simulink model "model_vec"  (R2022b)
settings: Solver=ode4  StartTime=0.0  StopTime=1.3  FixedStep=10e-6  RelTol=1e-3
InitFcn:
  | model_
values from neighbouring files (symbols this model uses):
  f = 50    [model_.m]
  i1dn = psi2n/Lm    [model_.m]
  i1qn = sqrt(Inmax^2-i1dn^2)    [model_.m]
  J = 0.4    [model_.m]
  L1 = L1sigma+Lm    (= 0.08477)    [model_.m]
  L1sigma = 2.27e-3    (= 0.00227)    [model_.m]
  L2 = L2sigma+Lm    (= 0.08477)    [model_.m]
  L2sigma = 2.27e-3    (= 0.00227)    [model_.m]
  Lm = 82.5e-3    (= 0.0825)    [model_.m]
  pp = 2    [model_.m]
  psi2n = sqrt(psi2nre^2+psi2nim^2)    [model_.m]
  R1 = 370e-3    (= 0.37)    [model_.m]
  R2 = 225e-3    (= 0.225)    [model_.m]
  R2_vec_model = 225e-3    (= 0.225)    [model_.m]
  sigma = 1-Lm^(2)/(L1*L2)    (= 0.0528396032209)    [model_.m]
  svmFrequency = 10000    [model_.m]
  Us = 400    [model_.m]
libraries: eeTransforms x16, spsMeanLib x7, slpidlib x4, simulink x2, dspsigops x2
(part 2 of 3)

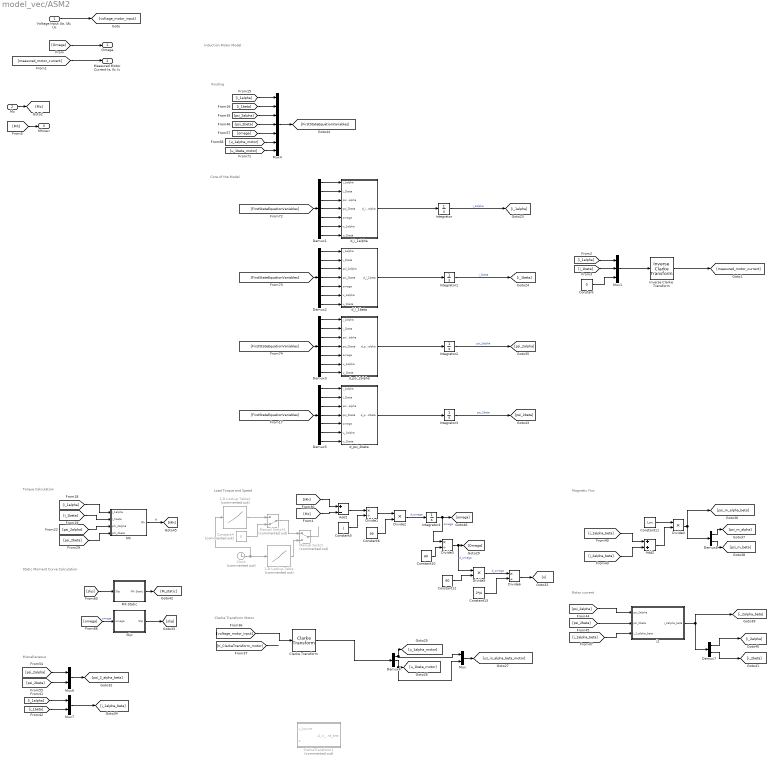
== system model_vec/ASM2 ==
  note: Clarke Transform Motor
  note: Induction Motor Model
  note: Rotor current
  note: Magnetic flux
  note: Static Moment Curve Calculation
  note: Routing
  note: Miscellaneous
  note: Load Torque and Speed
  note: Torque Calculation
  note: Core of the Model
  "Voltage Input Ua, Ub, Uc" : Inport
  Mz : Inport  Port=2
  1-D Lookup Table : Lookup_n-D  Commented=on  NumberOfTableDimensions=1  BreakpointsForDimension1=[0;1.00001;1.001;10]  Table=[0;0;25;25]  InternalRulePriority=Speed  RndMeth=Simplest
  1-D Lookup Table2 : Lookup_n-D  Commented=on  NumberOfTableDimensions=1  BreakpointsForDimension1=[1;2;10]  Table=[0;0;78.48]  InternalRulePriority=Speed  RndMeth=Simplest
  Add1 : Sum  Inputs=+-
  Add2 : Sum
  Clarke Transform : eeTransforms/Clarke Transform  PowerInvariant=off
      settings: LibrarySourceBlock=|
      | ee_sl_lib/Mathematical
      | Transforms/Clarke Transform
  ClarkeTransform1 : Subsystem  Commented=on
  Clock : Clock  Commented=on
  Constant : Constant  Value=0
  Constant10 : Constant  Value=pp
  Constant11 : Constant  Value=Lm
  Constant12 : Constant  Value=60
  Constant13 : Constant  Value=2*pi
  Constant4 : Constant  Commented=on  Value=0
  Constant5 : Constant  Value=J
  Constant6 : Constant  Value=pp
  Demux{1..3,5} (4 alike) : Demux  Outputs=7
  Demux6 : Demux  Outputs=3
  Demux7 : Demux  Outputs=2
  Demux8 : Demux  Outputs=2
  Divide1 : Product  Inputs=*/
  Divide2 : Product  Inputs=**
  Divide3 : Product  Inputs=*/
  Divide4 : Product  Inputs=**
  Divide5 : Product  Inputs=**
  Divide6 : Product  Inputs=*/
  Integrator{,1..4} (5 alike) : Integrator
  Inverse Clarke Transform : eeTransforms/Inverse Clarke Transform  PowerInvariant=off
      settings: LibrarySourceBlock=|
      | ee_sl_lib/Mathematical
      | Transforms/Inverse
      | Clarke Transform
  Manual Switch : ManualSwitch  Commented=on
  Manual Switch1 : ManualSwitch  Commented=on  CurrentSetting=0
  Mh : Subsystem
  Mh Static : Subsystem
  Mux : Mux  Inputs=2
  Mux1 : Mux  Inputs=3
  Mux4 : Mux  Inputs=7
  Mux6 : Mux  Inputs=2
  Mux7 : Mux  Inputs=2
  Slip : Subsystem
  d_i_1alpha : Subsystem
  d_i_1beta : Subsystem
  d_psi_2alpha : Subsystem
  d_psi_2beta : Subsystem
  i2 : Subsystem
  Omega : Outport
  "Measured Motor Current Ia, Ib, Ic" : Outport  Port=2
  Mhnaci : Outport  Port=3
  wires:
  "Voltage Input Ua, Ub, Uc"/1 -> [voltage_motor_input]
  [Omega] -> Omega/1
  [measured_motor_current] -> "Measured Motor Current Ia, Ib, Ic"/1
  Demux1/7 -> d_i_1alpha/7(u_1beta)
  [omega] -> Mux4/5
  Constant6/1 -> Divide2/2
  Demux7/2 -> [i_2beta]
  Constant13/1 -> Divide6/2
  Demux2/3 -> d_i_1beta/3(psi_2alpha)
  [K_ClarkeTransform_motor] -> ?
  1-D Lookup Table2/1 -> Manual Switch1/1
  [i_1alpha_beta] -> i2/3(i_1_alpha_beta)
  d_i_1alpha/1(d_i_1alpha) -> Integrator/1
  Constant4/1 -> Manual Switch1/2
  d_i_1beta/1(d_i_1beta) -> Integrator1/1
  Mh/1(Mh) -> [Mh]  "M"
  Divide6/1 -> [n]
  Demux3/5 -> d_psi_2alpha/5(omega)
  Demux1/2 -> d_i_1alpha/2(i_1beta)
  [i_1alpha] -> Mux7/1
  [psi_2alpha] -> Mh/3(phi_2alpha)
  Demux1/6 -> d_i_1alpha/6(u_1alpha)
  Demux5/7 -> d_psi_2beta/7(u_1beta)
  Demux5/1 -> d_psi_2beta/1(i_1alpha)
  i2/1(i_2alpha_beta) -> Demux7/1, [i_2alpha_beta]
  [i_1beta] -> Mux4/2
  Add2/1 -> Divide4/2
  Slip/1(Slip) -> [slip]
  Demux1/1 -> d_i_1alpha/1(i_1alpha)
  Constant5/1 -> Divide1/2
  Demux3/1 -> d_psi_2alpha/1(i_1alpha)
  Mux4/1 -> [FirstStateEquationVariables]
  [FirstStateEquationVariables] -> Demux5/1
  Integrator4/1 -> Divide3/1, [omega]  "omega"
  Manual Switch1/1 -> Manual Switch/1
  Constant10/1 -> Divide3/2
  Demux3/4 -> d_psi_2alpha/4(psi_2beta)
  Demux7/1 -> [i_2alpha]
  Add1/1 -> Divide1/1
  Demux5/5 -> d_psi_2beta/5(omega)
  [Mh] -> Add1/1
  Demux5/4 -> d_psi_2beta/4(psi_2beta)
  d_psi_2beta/1(d_psi_2beta) -> Integrator3/1
  [u_1beta_motor] -> Mux4/7
  Demux8/1 -> [psi_m_alpha]
  [i_1alpha_beta] -> Add2/1
  [i_1alpha] -> Mh/1(i_1alpha)
  Demux1/5 -> d_i_1alpha/5(omega)
  Demux2/6 -> d_i_1beta/6(u_1alpha)
  Demux2/2 -> d_i_1beta/2(i_1beta)
  Mux7/1 -> [i_1alpha_beta]
  [psi_2beta] -> i2/2(psi_2beta)
  Integrator2/1 -> [psi_2alpha]  "psi_2alpha"
  Demux1/4 -> d_i_1alpha/4(psi_2beta)
  Mux6/1 -> [psi_2_alpha_beta]
  [psi_2beta] -> Mh/4(phi_2beta)
  Constant12/1 -> Divide5/2
  1-D Lookup Table/1 -> Manual Switch/2
  Demux6/2 -> Mux/2, [u_1beta_motor]
  Demux3/3 -> d_psi_2alpha/3(psi_2alpha)
  [psi_2beta] -> Mux4/4
  Demux2/4 -> d_i_1beta/4(psi_2beta)
  [i_1beta] -> Mh/2(i_1beta)
  Divide1/1 -> Divide2/1
  Demux5/6 -> d_psi_2beta/6(u_1alpha)
  Demux2/1 -> d_i_1beta/1(i_1alpha)
  [i_2alpha_beta] -> Add2/2
  d_psi_2alpha/1(d_psi_2alpha) -> Integrator2/1
  Manual Switch/1 -> ?
  Divide2/1 -> Integrator4/1  "d_omega"
  [psi_2beta] -> Mux6/2
  Demux5/2 -> d_psi_2beta/2(i_1beta)
  Demux6/1 -> [u_1alpha_motor], Mux/1
  Divide3/1 -> Divide5/1, [Omega]  "d_omega"
  Integrator1/1 -> [i_1beta]  "i_1beta"
  Integrator3/1 -> [psi_2beta]  "psi_2beta"
  [i_1beta] -> Mux7/2
  Constant11/1 -> Divide4/1
  Demux2/5 -> d_i_1beta/5(omega)
  Demux8/2 -> [psi_m_beta]
  Demux3/6 -> d_psi_2alpha/6(u_1alpha)
  [FirstStateEquationVariables] -> Demux1/1
  Integrator/1 -> [i_1alpha]  "i_1alpha"
  [u_1alpha_motor] -> Mux4/6
  [FirstStateEquationVariables] -> Demux3/1
  [psi_2alpha] -> Mux4/3
  [psi_2alpha] -> i2/1(psi_2alpha)
  Divide5/1 -> Divide6/1  "d_omega"
  Demux2/7 -> d_i_1beta/7(u_1beta)
  Demux3/7 -> d_psi_2alpha/7(u_1beta)
  [slip] -> Mh Static/1(Slip)
  Demux3/2 -> d_psi_2alpha/2(i_1beta)
  Demux1/3 -> d_i_1alpha/3(psi_2alpha)
  [voltage_motor_input] -> Clarke Transform/1
  [FirstStateEquationVariables] -> Demux2/1
  Mh Static/1(Mh Static) -> [M_static]
  [psi_2alpha] -> Mux6/1
  [i_1alpha] -> Mux4/1
  [omega] -> Slip/1(omega)  "omega"
  Clock/1 -> 1-D Lookup Table2/1, 1-D Lookup Table/1
  Demux5/3 -> d_psi_2beta/3(psi_2alpha)
  Divide4/1 -> Demux8/1, [psi_m_alpha_beta]
  Clarke Transform/1 -> Demux6/1
  Mux/1 -> [u1_in_alpha_beta_motor]
  [i_1alpha] -> Mux1/1
  [i_1beta] -> Mux1/2
  Constant/1 -> Mux1/3
  Mux1/1 -> Inverse Clarke Transform/1
  Inverse Clarke Transform/1 -> [measured_motor_current]
  Mz/1 -> [Mz]
  [Mh] -> Mhnaci/1
  [Mz] -> Add1/2

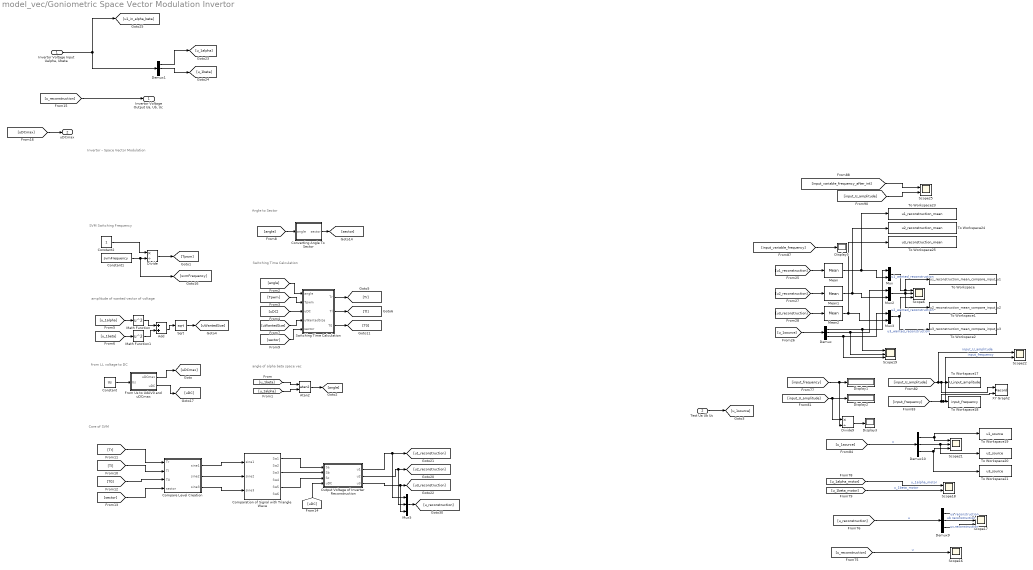
== system model_vec/Goniometric Space Vector Modulation Invertor ==
  note: Invertor – Space Vector Modulation
  note: Core of SVM
  note: Angle to Sector
  note: amplitude of wanted vector of voltage
  note: SVM Switching Frequency
  note: from LL voltage to DC
  note: Switching Time Calculation
  note: angle of alpha beta space vec
  "Invertor Voltage Input Ualpha, Ubeta" : Inport
  Test Ua Ub Uc : Inport  Port=2
  Add : Sum
  Atan2 : Trigonometry  Operator=atan2
  Comparation of Signal with Triangle Wave : Subsystem
  Compare Level Creation : Subsystem
  Constant : Constant  Value=Us
  Constant1 : Constant  Value=svmFrequency
  Constant2 : Constant
  Converting Angle To Sector : MATLAB Function  TreatAsAtomicUnit=on
  Demux{,1,9..10} (4 alike) : Demux  Outputs=3
  Display{1..3,5} (4 alike) : Display
  Divide : Product  Inputs=*/
  Divide9 : Product  Inputs=*/
  From Us to UdAV0 and uDCmax : MATLAB Function  TreatAsAtomicUnit=on
  Math Function : Math  Operator=square
  Math Function1 : Math  Operator=square
  Mean : spsMeanLib/Mean  Freq=svmFrequency  Vinit=0  Ts=0
  Mean1 : spsMeanLib/Mean  Freq=svmFrequency  Vinit=0  Ts=0
  Mean2 : spsMeanLib/Mean  Freq=svmFrequency  Vinit=0  Ts=0
  Mux : Mux  Inputs=2
  Mux2 : Mux  Inputs=2
  Mux3 : Mux  Inputs=2
  Mux5 : Mux  Inputs=3
  Output Voltage of Inverter Reconstruction : Subsystem
  Scope16 : Scope
  Scope{6,17,19,21} (4 alike) : Scope  NumInputPorts=3
  Scope18 : Scope  NumInputPorts=2
  Scope22 : Scope  NumInputPorts=2
  Scope25 : Scope  NumInputPorts=2
  Sqrt : Sqrt
  Switching Time Calculation : MATLAB Function  TreatAsAtomicUnit=on
  To Workspace : ToWorkspace  VariableName=u1_reconstruction_mean_compare_input_u1  SaveFormat=Timeseries  SampleTime=-1
  To Workspace1 : ToWorkspace  VariableName=u2_reconstruction_mean_compare_input_u2  SaveFormat=Timeseries  SampleTime=-1
  To Workspace17 : ToWorkspace  VariableName=U_input_amplitude  SaveFormat=Timeseries  SampleTime=-1
  To Workspace18 : ToWorkspace  VariableName=input_frequency  SaveFormat=Timeseries  SampleTime=-1
  To Workspace19 : ToWorkspace  VariableName=u1_source  SaveFormat=Timeseries  SampleTime=-1
  To Workspace2 : ToWorkspace  VariableName=u3_reconstruction_mean_compare_input_u3  SaveFormat=Timeseries  SampleTime=-1
  To Workspace20 : ToWorkspace  VariableName=u2_source  SaveFormat=Timeseries  SampleTime=-1
  To Workspace21 : ToWorkspace  VariableName=u3_source  SaveFormat=Timeseries  SampleTime=-1
  To Workspace23 : ToWorkspace  VariableName=u1_reconstruction_mean  SaveFormat=Timeseries  SampleTime=-1
  To Workspace24 : ToWorkspace  VariableName=u2_reconstruction_mean  SaveFormat=Timeseries  SampleTime=-1
  To Workspace25 : ToWorkspace  VariableName=u3_reconstruction_mean  SaveFormat=Timeseries  SampleTime=-1
  XY Graph2 : Record  FileSettingsInternal="{\"entries\":[{\"content\":{\"excelSettings\":{\"content\":{},\"type\":\"Streamout.ExcelSettings\"}},\"type\":\"Streamout.FileSettingStorage\",\"uuid\":\"02ea5c6f-de8f-4b43-b0a6-6bc7c7bf4af1\"}],\"packageUris\":[\"http://schema.mathworks.com/mf0/streamout_blocks/R2020a\"],\"version\":\"1.0\"}"  Layout=[1 1]  SignalsInternal="{\"entries\":[{\"content\":{\"signals\":[{\"content\":{\"blockPath\":[\"model_vec/Goniometric Space Vector Modulation Invertor/XY Graph2\"],\"channel\":[],\"dimensions\":[1],\"domain\":\"model_vec/Goniometric Space Vector Modulation Invertor/XY Graph2\",\"lineColor\":\"#0072bd\",\"plots\":[],\"port\":1,\"sid\":[\"\"],\"signalID\":2164,\"signalName\":\"input_U_amplitude\"},\"type\":\"RecordBlkView.Signal\",\"uuid\":\"30d02a87-ee14-4616-b6b9-5fcb510cce3f\"},{\"content\":{\"blockPath\":[\"model_vec/Goniometric Space Vector Modulation Invertor/XY Graph2\"],\"channel\":[],\"dimensions\":[1],\"domain\":\"model_vec/Goniometric Space Vector Modulation Invertor/XY Graph2\",\"lineColor\":\"#d95319\",\"plots\":[],\"port\":2,\"sid\":[\"\"],\"signalID\":2168,\"signalName\":\"input_frequency\"},\"type\":\"RecordBlkView.Signal\",\"uuid\":\"35793a4a-81a6-485c-847a-b82e39ee9c73\"}]},\"type\":\"RecordBlkView.InputSignals\",\"uuid\":\"5b8892b0-9142-4253-8381-be57873c5d0a\"}],\"packageUris\":[\"http://schema.mathworks.com/mf0/streamout_blocks/R2020a\"],\"version\":\"1.0\"}"  VisualizationBindings="{\"xyplotplugin\":{\"info\":[{\"series\":[],\"subplotID\":1}]}}"  CompatibilityTag=XY
  "Invertor Voltage Output Ua, Ub, Uc" : Outport
  uDCmax : Outport  Port=2
  wires:
  "Invertor Voltage Input Ualpha, Ubeta"/1 -> Demux1/1, [u1_in_alpha_beta]
  [u_reconstruction] -> "Invertor Voltage Output Ua, Ub, Uc"/1
  Demux1/1 -> [u_1alpha]
  Demux1/2 -> [u_1beta]
  [uDCmax] -> uDCmax/1
  Output Voltage of Inverter Reconstruction/3(u3) -> Mux5/3, [u3_reconstruction]
  [u_1beta] -> Atan2/1
  From Us to UdAV0 and uDCmax/1(uDCmax) -> [uDCmax]
  Divide/1 -> [Tpwm]
  [angle] -> Switching Time Calculation/1(angle)
  Converting Angle To Sector/1(sector) -> [sector]
  Atan2/1 -> [angle]
  [angle] -> Converting Angle To Sector/1(angle)
  Constant1/1 -> [svmFrequency], Divide/2
  [sector] -> Compare Level Creation/4(sector)
  Math Function/1 -> Add/1
  [Tr] -> Compare Level Creation/1(Tr)
  [uDC] -> Output Voltage of Inverter Reconstruction/4(uDC)
  [u_1alpha] -> Math Function/1
  [u_1alpha] -> Atan2/2
  [Tl] -> Compare Level Creation/2(Tl)
  Add/1 -> Sqrt/1
  [sector] -> Switching Time Calculation/5(sector)
  Constant/1 -> From Us to UdAV0 and uDCmax/1(Us)
  Output Voltage of Inverter Reconstruction/2(u2) -> Mux5/2, [u2_reconstruction]
  [Tpwm] -> Switching Time Calculation/2(Tpwm)
  Compare Level Creation/3(sine3) -> Comparation of Signal with Triangle Wave/3(sine3)
  Switching Time Calculation/3(T0) -> [T0]
  Comparation of Signal with Triangle Wave/3(Sw3) -> Output Voltage of Inverter Reconstruction/2(Sb)
  Comparation of Signal with Triangle Wave/5(Sw5) -> Output Voltage of Inverter Reconstruction/3(Sc)
  Output Voltage of Inverter Reconstruction/1(u1) -> Mux5/1, [u1_reconstruction]
  Compare Level Creation/1(sine1) -> Comparation of Signal with Triangle Wave/1(sine1)
  [uDC] -> Switching Time Calculation/3(uDC)
  Mux5/1 -> [u_reconstruction]
  From Us to UdAV0 and uDCmax/2(uDC) -> [uDC]
  [u_1beta] -> Math Function1/1
  Comparation of Signal with Triangle Wave/1(Sw1) -> Output Voltage of Inverter Reconstruction/1(Sa)
  Compare Level Creation/2(sine2) -> Comparation of Signal with Triangle Wave/2(sine2)
  Constant2/1 -> Divide/1
  Math Function1/1 -> Add/2
  [uWantedSize] -> Switching Time Calculation/4(uWantedSize)
  Switching Time Calculation/1(Tr) -> [Tr]
  Sqrt/1 -> [uWantedSize]
  [T0] -> Compare Level Creation/3(T0)
  Switching Time Calculation/2(Tl) -> [Tl]
  Divide9/1 -> Display3/1
  Mux3/1 -> Scope6/3, To Workspace2/1  "u3_wanted_reconstruction"
  [input_variable_frequency_after_int] -> Scope25/1
  [input_U_amplitude] -> Scope25/2
  Demux10/2 -> To Workspace20/1, Scope21/2
  Demux/1 -> Scope19/1, Mux/1
  [u_reconstruction] -> Demux9/1  "u"
  Mean2/1 -> To Workspace25/1, Mux3/2
  Demux10/3 -> To Workspace21/1, Scope21/3
  Demux/3 -> Scope19/3, Mux3/1
  Demux10/1 -> Scope21/1, To Workspace19/1
  [input_frequency] -> Scope22/2, To Workspace18/1, XY Graph2/2  "input_frequency"
  Demux/2 -> Scope19/2, Mux2/1
  [input_U_amplitude] -> Divide9/1, Display2/1
  [input_U_amplitude] -> Scope22/1, XY Graph2/1, To Workspace17/1  "input_U_amplitude"
  [u_1source] -> Demux10/1  "u"
  Mux/1 -> Scope6/1, To Workspace/1  "u1_wanted_reconstruction"
  Mean/1 -> To Workspace23/1, Mux/2
  [input_variable_frequency] -> Display5/1
  [u1_reconstruction] -> Mean/1
  [u3_reconstruction] -> Mean2/1
  Mux2/1 -> Scope6/2, To Workspace1/1  "u2_wanted_reconstruction"
  Mean1/1 -> To Workspace24/1, Mux2/2
  [input_frequency] -> Divide9/2, Display1/1
  [u2_reconstruction] -> Mean1/1
  Demux9/2 -> Scope17/2  "ub reconstruction"
  [u_reconstruction] -> Scope16/1  "u"
  [u_1alpha_motor] -> Scope18/1  "u_1alpha_motor"
  [u_1beta_motor] -> Scope18/2  "u_1beta_motor"
  [u_1source] -> Demux/1
  Demux9/1 -> Scope17/1  "ua reconstruction"
  Demux9/3 -> Scope17/3  "uc reconstruction"
  Test Ua Ub Uc/1 -> [u_1source]

== system model_vec/I-n model ==
  "Measured Motor Current Ia, Ib, Ic" : Inport
  Omega : Inport  Port=2
  Add : Sum  Inputs=+--
  Add1 : Sum  Inputs=+-+
  Atan2 : Trigonometry  Operator=atan2
  Clarke Transform : eeTransforms/Clarke Transform  PowerInvariant=off
      settings: LibrarySourceBlock=|
      | ee_sl_lib/Mathematical
      | Transforms/Clarke Transform
  Constant10 : Constant  Value=Lm
  Constant{7,9,11..12} (4 alike) : Constant  Value=L2
  Constant{2,5,13..14} (4 alike) : Constant  Value=R2_vec_model
  Constant4 : Constant  Value=pp
  Constant8 : Constant  Value=Lm
  Demux : Demux  Outputs=3
  Divide{,1..6} (7 alike) : Product  Inputs=**
  Divide10 : Product  Inputs=*/
  Divide7 : Product  Inputs=*/
  Divide8 : Product  Inputs=**/
  Divide9 : Product  Inputs=**/
  Integrator : Integrator
  Integrator1 : Integrator
  Module of Vector1 : Subsystem
  Mux : Mux  Inputs=2
  Theta : Outport
  Psi_2_module : Outport  Port=2
  Psi_2_alpha_beta : Outport  Port=3
  wires:
  "Measured Motor Current Ia, Ib, Ic"/1 -> Clarke Transform/1
  Clarke Transform/1 -> Demux/1
  Integrator1/1 -> [Psi_2_beta]  "Psi2beta"
  Demux/1 -> Divide/1  "i_1_alpha"
  Demux/2 -> Divide3/1  "i_1_beta"
  [omega] -> Divide2/1
  Integrator/1 -> [Psi_2_alpha]  "Psi2alpha"
  [Psi_2_beta] -> Divide2/2
  [Psi_2_alpha] -> Divide1/1
  Divide/1 -> Add/1
  Divide1/1 -> Add/2
  Divide2/1 -> Add/3
  Add/1 -> Integrator/1
  [Psi_2_beta] -> Divide4/1
  [Psi_2_alpha] -> Divide5/2
  [omega] -> Divide5/1
  Divide3/1 -> Add1/1
  Divide4/1 -> Add1/2
  Divide5/1 -> Add1/3
  Add1/1 -> Integrator1/1
  [Psi_2_beta] -> Atan2/1
  [Psi_2_alpha] -> Atan2/2
  Atan2/1 -> Theta/1
  [Psi_2_alpha] -> Mux/1, Module of Vector1/1(In1)
  [Psi_2_beta] -> Mux/2, Module of Vector1/2(In2)
  Module of Vector1/1(Psi) -> Psi_2_module/1  "psi_2_module"
  Omega/1 -> Divide6/1
  Constant4/1 -> Divide6/2
  Divide6/1 -> [omega]
  Mux/1 -> Psi_2_alpha_beta/1
  Divide7/1 -> Divide1/2
  Constant13/1 -> Divide7/1
  Constant7/1 -> Divide7/2
  Constant8/1 -> Divide8/1
  Constant5/1 -> Divide8/2
  Constant9/1 -> Divide8/3
  Divide8/1 -> Divide/2
  Constant11/1 -> Divide9/3
  Constant14/1 -> Divide9/2
  Constant10/1 -> Divide9/1
  Divide9/1 -> Divide3/2
  Constant12/1 -> Divide10/2
  Constant2/1 -> Divide10/1
  Divide10/1 -> Divide4/2

== system model_vec/Inverse Park1 ==
  dq0 : Inport
  Theta : Inport  Port=2
  Add : Sum  Inputs=+-
  Add1 : Sum
  Constant : Constant  Value=0
  Cos : Trigonometry  Operator=cos
  Cos1 : Trigonometry  Operator=cos
  Demux : Demux  Outputs=3
  Divide{,1..3} (4 alike) : Product  Inputs=**
  Mux : Mux  Inputs=3
  Sin : Trigonometry
  Sin1 : Trigonometry
  alpha_beta_0 : Outport
  wires:
  Constant/1 -> Mux/3
  Mux/1 -> alpha_beta_0/1
  Add1/1 -> Mux/2
  Add/1 -> Mux/1
  Divide2/1 -> Add1/2
  Divide3/1 -> Add1/1
  Divide/1 -> Add/2
  Divide1/1 -> Add/1
  [Theta] -> Cos1/1
  [Theta] -> Sin1/1
  Sin1/1 -> Divide2/1
  Cos1/1 -> Divide3/1
  [q] -> Divide3/2
  [d] -> Divide2/2
  [q] -> Divide/2
  [d] -> Divide1/2
  Demux/2 -> [q]
  Demux/1 -> [d]
  Cos/1 -> Divide1/1
  Sin/1 -> Divide/1
  [Theta] -> Sin/1
  [Theta] -> Cos/1
  Theta/1 -> [Theta]
  dq0/1 -> Demux/1

== system model_vec/Min-Max Method Space Vector Modulation Invertor ==
  note: from LL voltage to DC
  Ua Ub Uc : Inport
  Add12 : Sum
  Add13 : Sum  Inputs=+-
  Add14 : Sum  Inputs=+-
  Add15 : Sum  Inputs=+-
  Comparation of Signal with Triangle Wave : Subsystem
  Constant : Constant  Value=Us
  Constant13 : Constant  Value=270
  Constant14 : Constant  Value=2
  Demux : Demux  Outputs=3
  Demux1 : Demux  Outputs=3
  Divide{1..2,10..11} (4 alike) : Product  Inputs=*/
  From Us to UdAV0 and uDCmax : MATLAB Function  TreatAsAtomicUnit=on
  Max2 : MinMax  Function=max
  Max3 : MinMax
  Mean : spsMeanLib/Mean  Freq=svmFrequency  Vinit=0  Ts=0
  Mean1 : spsMeanLib/Mean  Freq=svmFrequency  Vinit=0  Ts=0
  Mean2 : spsMeanLib/Mean  Freq=svmFrequency  Vinit=0  Ts=0
  Mux : Mux  Inputs=2
  Mux2 : Mux  Inputs=2
  Mux3 : Mux  Inputs=2
  Mux5 : Mux  Inputs=3
  Output Voltage of Inverter Reconstruction : Subsystem
  Scope1 : Scope  NumInputPorts=3
  Scope6 : Scope  NumInputPorts=3
  u_reconstruction : Outport
  wires:
  Max2/1 -> Add12/1
  Ua Ub Uc/1 -> Demux1/1, Demux/1, Max3/1, Max2/1
  Constant13/1 -> Divide2/2, Divide1/2, Divide11/2
  Add13/1 -> Divide11/1
  Max3/1 -> Add12/2
  Add12/1 -> Divide10/1
  Constant14/1 -> Divide10/2
  Divide10/1 -> Add15/2, Add13/2, Add14/2
  Demux/1 -> Add13/1
  Comparation of Signal with Triangle Wave/5(Sw5) -> Output Voltage of Inverter Reconstruction/3(Sc)
  From Us to UdAV0 and uDCmax/2(uDC) -> [uDC]
  Output Voltage of Inverter Reconstruction/1(u1) -> Mean/1, Mux5/1, [u1_reconstruction]
  Output Voltage of Inverter Reconstruction/2(u2) -> Mean1/1, Mux5/2, [u2_reconstruction]
  [uDC] -> Output Voltage of Inverter Reconstruction/4(uDC)
  Mux5/1 -> u_reconstruction/1
  From Us to UdAV0 and uDCmax/1(uDCmax) -> [uDCmax]
  Comparation of Signal with Triangle Wave/1(Sw1) -> Output Voltage of Inverter Reconstruction/1(Sa)
  Output Voltage of Inverter Reconstruction/3(u3) -> Mean2/1, Mux5/3, [u3_reconstruction]
  Constant/1 -> From Us to UdAV0 and uDCmax/1(Us)
  Comparation of Signal with Triangle Wave/3(Sw3) -> Output Voltage of Inverter Reconstruction/2(Sb)
  Demux/2 -> Add14/1
  Demux/3 -> Add15/1
  Divide11/1 -> Comparation of Signal with Triangle Wave/1(sine1), Scope6/1
  Add14/1 -> Divide1/1
  Add15/1 -> Divide2/1
  Divide1/1 -> Comparation of Signal with Triangle Wave/2(sine2), Scope6/2
  Divide2/1 -> Scope6/3, Comparation of Signal with Triangle Wave/3(sine3)
  Mean/1 -> Mux/1
  Mean1/1 -> Mux2/1
  Mean2/1 -> Mux3/1
  Mux/1 -> Scope1/1  "u1_wanted_reconstruction"
  Mux2/1 -> Scope1/2  "u2_wanted_reconstruction"
  Mux3/1 -> Scope1/3  "u3_wanted_reconstruction"
  Demux1/3 -> Mux3/2
  Demux1/2 -> Mux2/2
  Demux1/1 -> Mux/2

== system model_vec/Odvazbeni u1d (pricist k u1d) (minusy jsou uvnitr) ==
  i1q : Inport
  psi2d : Inport  Port=2
  omega_s : Inport  Port=3
  Add11 : Sum  Inputs=+-
  Add14 : Sum  Inputs=--
  Constant3 : Constant  Value=L1
  Constant5 : Constant  Value=Lm^2/L2
  Constant6 : Constant  Value=Lm*R2_vec_model/L2^2
  Divide : Product  Inputs=***
  Divide1 : Product  Inputs=**
  odvazbeni : Outport
  wires:
  Constant6/1 -> Divide1/1
  i1q/1 -> Divide/3
  Divide/1 -> Add14/1
  Add11/1 -> Divide/1
  psi2d/1 -> Divide1/2
  Constant5/1 -> Add11/2
  Add14/1 -> odvazbeni/1
  Constant3/1 -> Add11/1
  Divide1/1 -> Add14/2
  omega_s/1 -> Divide/2

== system model_vec/Odvazbeni u1q (pricist k u1q) (minusy jsou uvnitr) ==
  i1d : Inport
  psi2d : Inport  Port=2
  omega_s : Inport  Port=3
  Add11 : Sum  Inputs=+-
  Add14 : Sum
  Constant1 : Constant  Value=2*pi*f
  Constant2 : Constant  Value=Lm/L2
  Constant3 : Constant  Value=L1
  Constant5 : Constant  Value=Lm^2/L2
  Divide : Product  Inputs=***
  Divide1 : Product  Inputs=***
  odvazbeni : Outport
  wires:
  Divide1/1 -> Add14/2
  Constant3/1 -> Add11/1
  Add14/1 -> odvazbeni/1
  Constant5/1 -> Add11/2
  psi2d/1 -> Divide1/2
  Add11/1 -> Divide/1
  Divide/1 -> Add14/1
  i1d/1 -> Divide/3
  Constant1/1 -> Divide1/1
  Constant2/1 -> Divide1/3
  omega_s/1 -> Divide/2

== system model_vec/Omega*Time Calculation1 ==
  frequency : Inport
  Clock : Clock  Commented=on
  Constant1 : Constant  Commented=on  Value=50
  Constant2 : Constant  Commented=on
  Constant4 : Constant  Value=2
  Constant5 : Constant  Value=pi
  Divide1 : Product  Inputs=***
  Equal : RelationalOperator  Commented=on  OutDataTypeStr=boolean  RndMeth=Simplest  InputSameDT=off
  Switch : Switch  Commented=on  Criteria=u2 > Threshold  SaturateOnIntegerOverflow=off  InputSameDT=off
  omega_t : Outport
  wires:
  Divide1/1 -> omega_t/1
  frequency/1 -> Divide1/3
  Constant5/1 -> Divide1/2
  Clock/1 -> Switch/1
  Constant4/1 -> Divide1/1
  Constant1/1 -> Equal/2
  Equal/1 -> Switch/2
  Constant2/1 -> Switch/3

== system model_vec/Triggered Subsystem ==
  In1 : Inport
  Trigger : TriggerPort  VariantControl=(inherit)
  Out1 : Outport
  wires:
  In1/1 -> Out1/1

== system model_vec/u4 ==
  amplitude : Inport
  omega_t : Inport  Port=2
  Add4 : Sum
  Constant6 : Constant  Value=0
  Divide3 : Product  Inputs=**
  Sin : Trigonometry
  u1 : Outport
  wires:
  Divide3/1 -> u1/1
  Sin/1 -> Divide3/1
  Add4/1 -> Sin/1
  Constant6/1 -> Add4/2
  omega_t/1 -> Add4/1
  amplitude/1 -> Divide3/2

== system model_vec/u5 ==
  amplitude : Inport
  omega_t : Inport  Port=2
  Add4 : Sum
  Constant6 : Constant  Value=(2*pi/3)
  Divide3 : Product  Inputs=**
  Sin : Trigonometry
  u2 : Outport
  wires:
  omega_t/1 -> Add4/1
  Constant6/1 -> Add4/2
  Add4/1 -> Sin/1
  Sin/1 -> Divide3/1
  Divide3/1 -> u2/1
  amplitude/1 -> Divide3/2

== system model_vec/u6 ==
  amplitude : Inport
  omega_t : Inport  Port=2
  Add4 : Sum
  Constant6 : Constant  Value=(-2*pi/3)
  Divide3 : Product  Inputs=**
  Sin : Trigonometry
  u3 : Outport
  wires:
  Divide3/1 -> u3/1
  amplitude/1 -> Divide3/2
  Sin/1 -> Divide3/1
  Add4/1 -> Sin/1
  Constant6/1 -> Add4/2
  omega_t/1 -> Add4/1

== system model_vec/ASM/ClarkeTransform1 ==
  u_1source : Inport
  K : Inport  Port=2
  Add1 : Sum  Inputs=+++
  Add2 : Sum  Inputs=+++
  Demux4 : Demux  Outputs=3
  Demux5 : Demux  Outputs=3
  Divide2 : Product  Inputs=**
  Divide3 : Product  Inputs=**
  Gain : Gain  Gain=-1/2
  Gain1 : Gain  Gain=-1/2
  Gain2 : Gain  Gain=-sqrt(3)/2
  Gain3 : Gain  Gain=sqrt(3)/2
  Gain4 : Gain
  Gain5 : Gain  Gain=0
  Mux2 : Mux  Inputs=2
  u1_in_alpha_beta : Outport
  wires:
  Demux4/1 -> Gain4/1  "ua"
  Divide2/1 -> Mux2/1  "u_1alpha"
  [K_ClarkeTransform] -> Divide2/2
  Add1/1 -> Divide2/1
  Demux4/2 -> Gain/1  "ub"
  Divide3/1 -> Mux2/2  "u_1beta"
  Gain5/1 -> Add2/1
  Gain/1 -> Add1/2
  Demux5/1 -> Gain5/1  "ua"
  Gain3/1 -> Add2/3
  [K_ClarkeTransform] -> Divide3/2
  Gain2/1 -> Add2/2
  Gain1/1 -> Add1/3
  Demux5/2 -> Gain2/1  "ub"
  Demux5/3 -> Gain3/1  "uc"
  Add2/1 -> Divide3/1
  Gain4/1 -> Add1/1
  u_1source/1 -> Demux5/1, Demux4/1
  K/1 -> [K_ClarkeTransform]
  Mux2/1 -> u1_in_alpha_beta/1
  Demux4/3 -> Gain1/1  "uc"

== system model_vec/ASM/Mh ==
  i_1alpha : Inport
  i_1beta : Inport  Port=2
  phi_2alpha : Inport  Port=3
  phi_2beta : Inport  Port=4
  Add : Sum  Inputs=+-
  Constant : Constant  Value=3/2
  Constant1 : Constant  Value=pp
  Constant2 : Constant  Value=Lm
  Constant3 : Constant  Value=L2
  Divide{,1,3..5} (5 alike) : Product  Inputs=**
  Divide2 : Product  Inputs=*/
  Mh : Outport
  wires:
  Constant/1 -> Divide/1
  Constant1/1 -> Divide/2
  Divide/1 -> Divide1/1
  Constant2/1 -> Divide2/1
  Constant3/1 -> Divide2/2
  Divide2/1 -> Divide1/2
  Divide1/1 -> Divide3/2
  phi_2alpha/1 -> Divide4/2
  i_1beta/1 -> Divide4/1
  Divide4/1 -> Add/1
  phi_2beta/1 -> Divide5/1
  i_1alpha/1 -> Divide5/2
  Divide5/1 -> Add/2
  Add/1 -> Divide3/1
  Divide3/1 -> Mh/1

== system model_vec/ASM/Mh Static ==
  Slip : Inport
  Add3 : Sum
  Add4 : Sum
  Add6 : Sum
  Constant10 : Constant  Value=230^(2)
  Constant11 : Constant  Value=pp
  Constant14 : Constant  Value=2*pi*f
  Constant15 : Constant  Value=R1
  Constant16 : Constant  Value=R2
  Constant21 : Constant  Value=2*pi*f
  Constant22 : Constant  Value=L1sigma
  Constant23 : Constant  Value=L2sigma
  Constant8 : Constant  Value=3
  Constant9 : Constant  Value=R2
  Divide10 : Product  Inputs=/*
  Divide11 : Product  Inputs=*/
  Divide15 : Product  Inputs=**
  Divide6 : Product  Inputs=****
  Divide7 : Product  Inputs=*/
  Divide8 : Product  Inputs=**
  Math Function : Math  Operator=square
  Math Function2 : Math  Operator=square
  Reprezentace s s*omega1*L2sigma : Subsystem
  Mh Static : Outport
  wires:
  Slip/1 -> Divide8/2, Divide11/2
  Constant11/1 -> Divide6/4
  Constant10/1 -> Divide6/3
  Add4/1 -> Math Function/1
  Constant16/1 -> Divide11/1
  Constant9/1 -> Divide6/2
  Constant23/1 -> Add6/2
  Constant15/1 -> Add4/1
  Divide15/1 -> Math Function2/1
  Divide8/1 -> Divide7/2
  Constant14/1 -> Divide8/1
  Math Function/1 -> Add3/1
  Divide7/1 -> Divide10/2
  Divide10/1 -> Mh Static/1
  Divide11/1 -> Add4/2
  Constant22/1 -> Add6/1
  Add6/1 -> Divide15/1
  Constant8/1 -> Divide6/1
  Constant21/1 -> Divide15/2
  Add3/1 -> Divide10/1
  Divide6/1 -> Divide7/1
  Math Function2/1 -> Add3/2

== system model_vec/ASM/Module of Vector ==
  In1 : Inport
  In2 : Inport  Port=2
  Add2 : Sum
  Math Function : Math  Operator=square
  Math Function1 : Math  Operator=square
  Sqrt : Sqrt
  Out1 : Outport
  wires:
  In1/1 -> Math Function/1
  Sqrt/1 -> Out1/1
  Math Function/1 -> Add2/1
  Math Function1/1 -> Add2/2
  In2/1 -> Math Function1/1
  Add2/1 -> Sqrt/1

== system model_vec/ASM/Module of Vector1 ==
  In1 : Inport
  In2 : Inport  Port=2
  Add2 : Sum
  Math Function : Math  Operator=square
  Math Function1 : Math  Operator=square
  Sqrt : Sqrt
  Out1 : Outport
  wires:
  Add2/1 -> Sqrt/1
  In2/1 -> Math Function1/1
  Math Function1/1 -> Add2/2
  Math Function/1 -> Add2/1
  Sqrt/1 -> Out1/1
  In1/1 -> Math Function/1

== system model_vec/ASM/Module of Vector2 ==
  In1 : Inport
  In2 : Inport  Port=2
  Add2 : Sum
  Math Function : Math  Operator=square
  Math Function1 : Math  Operator=square
  Sqrt : Sqrt
  Out1 : Outport
  wires:
  Add2/1 -> Sqrt/1
  In2/1 -> Math Function1/1
  Math Function1/1 -> Add2/2
  Math Function/1 -> Add2/1
  Sqrt/1 -> Out1/1
  In1/1 -> Math Function/1

== system model_vec/ASM/Slip ==
  omega : Inport
  Add2 : Sum  Inputs=+-
  Constant12 : Constant  Value=2*pi*f
  Constant13 : Constant  Value=2*pi*f
  Divide9 : Product  Inputs=*/
  Slip : Outport
  wires:
  omega/1 -> Add2/2  "Omega"
  Divide9/1 -> Slip/1
  Constant12/1 -> Add2/1
  Add2/1 -> Divide9/1
  Constant13/1 -> Divide9/2

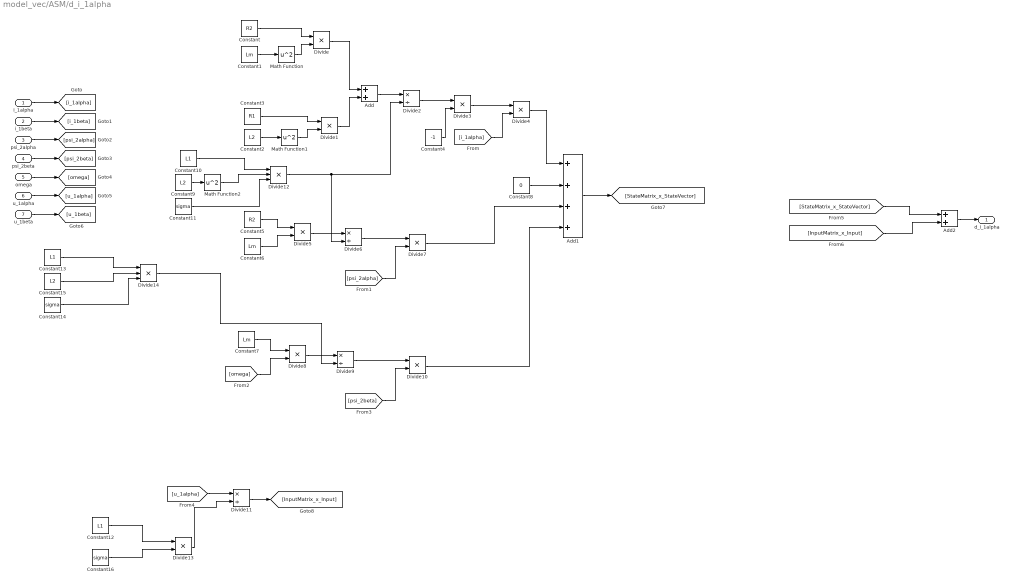
== system model_vec/ASM/d_i_1alpha ==
  i_1alpha : Inport
  i_1beta : Inport  Port=2
  psi_2alpha : Inport  Port=3
  psi_2beta : Inport  Port=4
  omega : Inport  Port=5
  u_1alpha : Inport  Port=6
  u_1beta : Inport  Port=7
  Add : Sum
  Add1 : Sum  Inputs=++++
  Add2 : Sum
  Constant : Constant  Value=R2
  Constant1 : Constant  Value=Lm
  Constant10 : Constant  Value=L1
  Constant11 : Constant  Value=sigma
  Constant12 : Constant  Value=L1
  Constant13 : Constant  Value=L1
  Constant14 : Constant  Value=sigma
  Constant15 : Constant  Value=L2
  Constant16 : Constant  Value=sigma
  Constant2 : Constant  Value=L2
  Constant3 : Constant  Value=R1
  Constant4 : Constant  Value=-1
  Constant5 : Constant  Value=R2
  Constant6 : Constant  Value=Lm
  Constant7 : Constant  Value=Lm
  Constant8 : Constant  Value=0
  Constant9 : Constant  Value=L2
  Divide{,1,3..5,7..8,10,13} (9 alike) : Product  Inputs=**
  Divide{2,6,9,11} (4 alike) : Product  Inputs=*/
  Divide12 : Product  Inputs=***
  Divide14 : Product  Inputs=***
  Math Function : Math  Operator=square
  Math Function1 : Math  Operator=square
  Math Function2 : Math  Operator=square
  d_i_1alpha : Outport
  wires:
  Constant1/1 -> Math Function/1
  Constant/1 -> Divide/1
  Math Function/1 -> Divide/2
  Divide/1 -> Add/1
  Constant2/1 -> Math Function1/1
  Constant3/1 -> Divide1/1
  Math Function1/1 -> Divide1/2
  Divide1/1 -> Add/2
  Add/1 -> Divide2/1
  Constant4/1 -> Divide3/2
  Divide2/1 -> Divide3/1
  Divide3/1 -> Divide4/1
  i_1alpha/1 -> [i_1alpha]
  i_1beta/1 -> [i_1beta]
  psi_2alpha/1 -> [psi_2alpha]
  psi_2beta/1 -> [psi_2beta]
  omega/1 -> [omega]
  [i_1alpha] -> Divide4/2
  Divide4/1 -> Add1/1
  Constant5/1 -> Divide5/1
  Constant6/1 -> Divide5/2
  Divide5/1 -> Divide6/1
  Divide6/1 -> Divide7/1
  [psi_2alpha] -> Divide7/2
  Divide7/1 -> Add1/3
  Constant7/1 -> Divide8/1
  [omega] -> Divide8/2
  Divide8/1 -> Divide9/1
  Divide9/1 -> Divide10/1
  [psi_2beta] -> Divide10/2
  Divide10/1 -> Add1/4
  Constant8/1 -> Add1/2
  u_1alpha/1 -> [u_1alpha]
  u_1beta/1 -> [u_1beta]
  Add1/1 -> [StateMatrix_x_StateVector]
  [u_1alpha] -> Divide11/1
  Divide11/1 -> [InputMatrix_x_Input]
  [StateMatrix_x_StateVector] -> Add2/1
  [InputMatrix_x_Input] -> Add2/2
  Add2/1 -> d_i_1alpha/1
  Constant9/1 -> Math Function2/1
  Constant10/1 -> Divide12/1
  Math Function2/1 -> Divide12/2
  Constant11/1 -> Divide12/3
  Divide12/1 -> Divide6/2, Divide2/2
  Constant14/1 -> Divide14/3
  Constant13/1 -> Divide14/1
  Constant15/1 -> Divide14/2
  Constant12/1 -> Divide13/1
  Constant16/1 -> Divide13/2
  Divide13/1 -> Divide11/2
  Divide14/1 -> Divide9/2

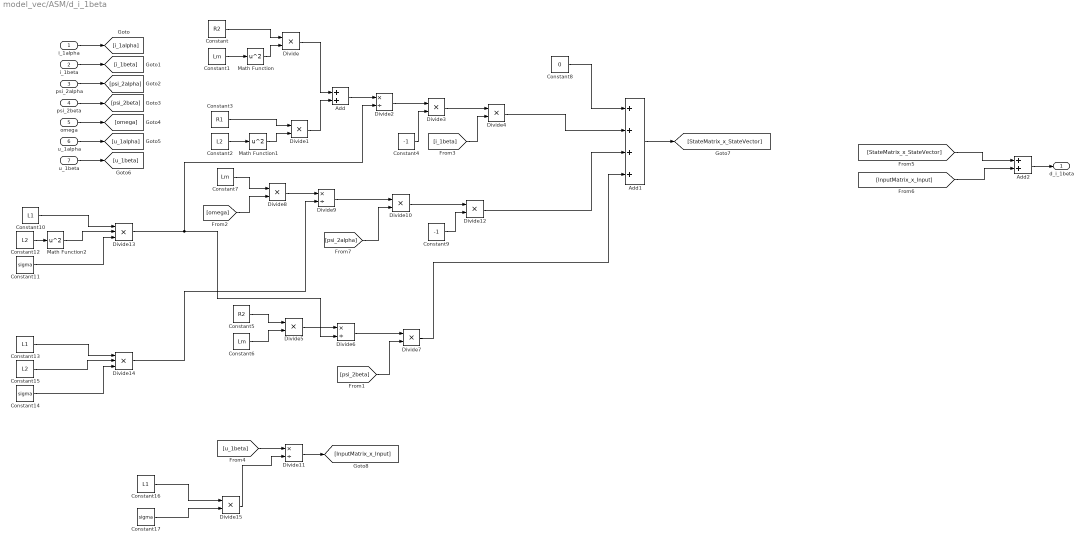
== system model_vec/ASM/d_i_1beta ==
  i_1alpha : Inport
  i_1beta : Inport  Port=2
  psi_2alpha : Inport  Port=3
  psi_2beta : Inport  Port=4
  omega : Inport  Port=5
  u_1alpha : Inport  Port=6
  u_1beta : Inport  Port=7
  Add : Sum
  Add1 : Sum  Inputs=++++
  Add2 : Sum
  Constant : Constant  Value=R2
  Constant1 : Constant  Value=Lm
  Constant10 : Constant  Value=L1
  Constant11 : Constant  Value=sigma
  Constant12 : Constant  Value=L2
  Constant13 : Constant  Value=L1
  Constant14 : Constant  Value=sigma
  Constant15 : Constant  Value=L2
  Constant16 : Constant  Value=L1
  Constant17 : Constant  Value=sigma
  Constant2 : Constant  Value=L2
  Constant3 : Constant  Value=R1
  Constant4 : Constant  Value=-1
  Constant5 : Constant  Value=R2
  Constant6 : Constant  Value=Lm
  Constant7 : Constant  Value=Lm
  Constant8 : Constant  Value=0
  Constant9 : Constant  Value=-1
  Divide{,1,3..5,7..8,10,12,15} (10 alike) : Product  Inputs=**
  Divide{2,6,9,11} (4 alike) : Product  Inputs=*/
  Divide13 : Product  Inputs=***
  Divide14 : Product  Inputs=***
  Math Function : Math  Operator=square
  Math Function1 : Math  Operator=square
  Math Function2 : Math  Operator=square
  d_i_1beta : Outport
  wires:
  Add2/1 -> d_i_1beta/1
  [InputMatrix_x_Input] -> Add2/2
  [StateMatrix_x_StateVector] -> Add2/1
  Divide11/1 -> [InputMatrix_x_Input]
  [u_1beta] -> Divide11/1
  Add1/1 -> [StateMatrix_x_StateVector]
  u_1beta/1 -> [u_1beta]
  u_1alpha/1 -> [u_1alpha]
  Constant8/1 -> Add1/1
  Divide10/1 -> Divide12/1
  [psi_2alpha] -> Divide10/2
  Divide9/1 -> Divide10/1
  Divide8/1 -> Divide9/1
  [omega] -> Divide8/2
  Constant7/1 -> Divide8/1
  Divide7/1 -> Add1/4
  [psi_2beta] -> Divide7/2
  Divide6/1 -> Divide7/1
  Divide5/1 -> Divide6/1
  Constant6/1 -> Divide5/2
  Constant5/1 -> Divide5/1
  Divide4/1 -> Add1/2
  [i_1beta] -> Divide4/2
  omega/1 -> [omega]
  psi_2beta/1 -> [psi_2beta]
  psi_2alpha/1 -> [psi_2alpha]
  i_1beta/1 -> [i_1beta]
  i_1alpha/1 -> [i_1alpha]
  Divide3/1 -> Divide4/1
  Divide2/1 -> Divide3/1
  Constant4/1 -> Divide3/2
  Add/1 -> Divide2/1
  Divide1/1 -> Add/2
  Math Function1/1 -> Divide1/2
  Constant3/1 -> Divide1/1
  Constant2/1 -> Math Function1/1
  Divide/1 -> Add/1
  Math Function/1 -> Divide/2
  Constant/1 -> Divide/1
  Constant1/1 -> Math Function/1
  Constant9/1 -> Divide12/2
  Divide12/1 -> Add1/3
  Constant10/1 -> Divide13/1
  Constant11/1 -> Divide13/3
  Math Function2/1 -> Divide13/2
  Divide13/1 -> Divide6/2, Divide2/2
  Constant12/1 -> Math Function2/1
  Divide14/1 -> Divide9/2
  Constant14/1 -> Divide14/3
  Constant15/1 -> Divide14/2
  Constant13/1 -> Divide14/1
  Constant16/1 -> Divide15/1
  Divide15/1 -> Divide11/2
  Constant17/1 -> Divide15/2

== system model_vec/ASM/d_psi_2alpha ==
  note: je to jen pro úplnost
  i_1alpha : Inport
  i_1beta : Inport  Port=2
  psi_2alpha : Inport  Port=3
  psi_2beta : Inport  Port=4
  omega : Inport  Port=5
  u_1alpha : Inport  Port=6
  u_1beta : Inport  Port=7
  Add1 : Sum  Inputs=++++
  Add2 : Sum
  Constant : Constant  Value=0
  Constant1 : Constant  Value=-1
  Constant2 : Constant  Value=-1
  Constant3 : Constant  Value=R2
  Constant4 : Constant  Value=L2
  Constant5 : Constant  Value=Lm
  Constant6 : Constant  Value=R2
  Constant7 : Constant  Value=L2
  Constant8 : Constant  Value=0
  Divide{,1,3..5,7} (6 alike) : Product  Inputs=**
  Divide2 : Product  Inputs=*/
  Divide6 : Product  Inputs=*/
  d_psi_2alpha : Outport
  wires:
  i_1alpha/1 -> [i_1alpha]
  i_1beta/1 -> [i_1beta]
  psi_2alpha/1 -> [psi_2alpha]
  psi_2beta/1 -> [psi_2beta]
  omega/1 -> [omega]
  Constant8/1 -> Add1/2
  u_1alpha/1 -> [u_1alpha]
  u_1beta/1 -> [u_1beta]
  Add1/1 -> [StateMatrix_x_StateVector]
  Constant/1 -> [InputMatrix_x_Input]
  [StateMatrix_x_StateVector] -> Add2/1
  [InputMatrix_x_Input] -> Add2/2
  Add2/1 -> d_psi_2alpha/1
  [omega] -> Divide/1
  Constant1/1 -> Divide/2
  Divide/1 -> Divide1/1
  [psi_2beta] -> Divide1/2
  Divide1/1 -> Add1/4
  Constant2/1 -> Divide3/2
  Divide2/1 -> Divide3/1
  Constant3/1 -> Divide2/1
  Constant4/1 -> Divide2/2
  Divide3/1 -> Divide4/1
  [psi_2alpha] -> Divide4/2
  Divide4/1 -> Add1/3
  Divide5/1 -> Divide6/1
  Constant5/1 -> Divide5/1
  Constant6/1 -> Divide5/2
  Constant7/1 -> Divide6/2
  Divide6/1 -> Divide7/1
  [i_1alpha] -> Divide7/2
  Divide7/1 -> Add1/1

== system model_vec/ASM/d_psi_2beta ==
  i_1alpha : Inport
  i_1beta : Inport  Port=2
  psi_2alpha : Inport  Port=3
  psi_2beta : Inport  Port=4
  omega : Inport  Port=5
  u_1alpha : Inport  Port=6
  u_1beta : Inport  Port=7
  Add1 : Sum  Inputs=++++
  Add2 : Sum
  Constant : Constant  Value=0
  Constant2 : Constant  Value=-1
  Constant3 : Constant  Value=R2
  Constant4 : Constant  Value=L2
  Constant5 : Constant  Value=Lm
  Constant6 : Constant  Value=R2
  Constant7 : Constant  Value=L2
  Constant8 : Constant  Value=0
  Divide{1,3..5,7} (5 alike) : Product  Inputs=**
  Divide2 : Product  Inputs=*/
  Divide6 : Product  Inputs=*/
  d_psi_2beta : Outport
  wires:
  Divide7/1 -> Add1/2
  [i_1beta] -> Divide7/2
  Divide6/1 -> Divide7/1
  Constant7/1 -> Divide6/2
  Constant6/1 -> Divide5/2
  Constant5/1 -> Divide5/1
  Divide5/1 -> Divide6/1
  Divide4/1 -> Add1/4
  [psi_2beta] -> Divide4/2
  Divide3/1 -> Divide4/1
  Constant4/1 -> Divide2/2
  Constant3/1 -> Divide2/1
  Divide2/1 -> Divide3/1
  Constant2/1 -> Divide3/2
  Divide1/1 -> Add1/3
  [psi_2alpha] -> Divide1/2
  Add2/1 -> d_psi_2beta/1
  [InputMatrix_x_Input] -> Add2/2
  [StateMatrix_x_StateVector] -> Add2/1
  Constant/1 -> [InputMatrix_x_Input]
  Add1/1 -> [StateMatrix_x_StateVector]
  u_1beta/1 -> [u_1beta]
  u_1alpha/1 -> [u_1alpha]
  Constant8/1 -> Add1/1
  omega/1 -> [omega]
  psi_2beta/1 -> [psi_2beta]
  psi_2alpha/1 -> [psi_2alpha]
  i_1beta/1 -> [i_1beta]
  i_1alpha/1 -> [i_1alpha]
  [omega] -> Divide1/1

== system model_vec/ASM/i2 ==
  psi_2alpha : Inport
  psi_2beta : Inport  Port=2
  i_1_alpha_beta : Inport  Port=3
  Add2 : Sum  Inputs=+-
  Constant6 : Constant  Value=Lm
  Constant7 : Constant  Value=L2
  Divide4 : Product  Inputs=**
  Divide5 : Product  Inputs=*/
  Mux2 : Mux  Inputs=2
  i_2alpha_beta : Outport
  wires:
  psi_2alpha/1 -> Mux2/1
  Mux2/1 -> Add2/1
  Add2/1 -> Divide5/1
  Constant6/1 -> Divide4/2
  Divide4/1 -> Add2/2
  psi_2beta/1 -> Mux2/2
  Constant7/1 -> Divide5/2
  Divide5/1 -> i_2alpha_beta/1
  i_1_alpha_beta/1 -> Divide4/1

== system model_vec/ASM1/ClarkeTransform1 ==
  u_1source : Inport
  K : Inport  Port=2
  Add1 : Sum  Inputs=+++
  Add2 : Sum  Inputs=+++
  Demux4 : Demux  Outputs=3
  Demux5 : Demux  Outputs=3
  Divide2 : Product  Inputs=**
  Divide3 : Product  Inputs=**
  Gain : Gain  Gain=-1/2
  Gain1 : Gain  Gain=-1/2
  Gain2 : Gain  Gain=-sqrt(3)/2
  Gain3 : Gain  Gain=sqrt(3)/2
  Gain4 : Gain
  Gain5 : Gain  Gain=0
  Mux2 : Mux  Inputs=2
  u1_in_alpha_beta : Outport
  wires:
  Demux4/3 -> Gain1/1  "uc"
  Mux2/1 -> u1_in_alpha_beta/1
  K/1 -> [K_ClarkeTransform]
  u_1source/1 -> Demux4/1, Demux5/1
  Gain4/1 -> Add1/1
  Add2/1 -> Divide3/1
  Demux5/3 -> Gain3/1  "uc"
  Demux5/2 -> Gain2/1  "ub"
  Gain1/1 -> Add1/3
  Gain2/1 -> Add2/2
  [K_ClarkeTransform] -> Divide3/2
  Gain3/1 -> Add2/3
  Demux5/1 -> Gain5/1  "ua"
  Gain/1 -> Add1/2
  Gain5/1 -> Add2/1
  Divide3/1 -> Mux2/2  "u_1beta"
  Demux4/2 -> Gain/1  "ub"
  Add1/1 -> Divide2/1
  [K_ClarkeTransform] -> Divide2/2
  Divide2/1 -> Mux2/1  "u_1alpha"
  Demux4/1 -> Gain4/1  "ua"

== system model_vec/ASM1/Mh ==
  i_1alpha : Inport
  i_1beta : Inport  Port=2
  phi_2alpha : Inport  Port=3
  phi_2beta : Inport  Port=4
  Add : Sum  Inputs=+-
  Constant : Constant  Value=3/2
  Constant1 : Constant  Value=pp
  Constant2 : Constant  Value=Lm
  Constant3 : Constant  Value=L2
  Divide{,1,3..5} (5 alike) : Product  Inputs=**
  Divide2 : Product  Inputs=*/
  Mh : Outport
  wires:
  Divide3/1 -> Mh/1
  Add/1 -> Divide3/1
  Divide5/1 -> Add/2
  i_1alpha/1 -> Divide5/2
  phi_2beta/1 -> Divide5/1
  Divide4/1 -> Add/1
  i_1beta/1 -> Divide4/1
  phi_2alpha/1 -> Divide4/2
  Divide1/1 -> Divide3/2
  Divide2/1 -> Divide1/2
  Constant3/1 -> Divide2/2
  Constant2/1 -> Divide2/1
  Divide/1 -> Divide1/1
  Constant1/1 -> Divide/2
  Constant/1 -> Divide/1

== system model_vec/ASM1/Mh Static ==
  Slip : Inport
  Add3 : Sum
  Add4 : Sum
  Add6 : Sum
  Constant10 : Constant  Value=230^(2)
  Constant11 : Constant  Value=pp
  Constant14 : Constant  Value=2*pi*f
  Constant15 : Constant  Value=R1
  Constant16 : Constant  Value=R2
  Constant21 : Constant  Value=2*pi*f
  Constant22 : Constant  Value=L1sigma
  Constant23 : Constant  Value=L2sigma
  Constant8 : Constant  Value=3
  Constant9 : Constant  Value=R2
  Divide10 : Product  Inputs=/*
  Divide11 : Product  Inputs=*/
  Divide15 : Product  Inputs=**
  Divide6 : Product  Inputs=****
  Divide7 : Product  Inputs=*/
  Divide8 : Product  Inputs=**
  Math Function : Math  Operator=square
  Math Function2 : Math  Operator=square
  Reprezentace s s*omega1*L2sigma : Subsystem
  Mh Static : Outport
  wires:
  Math Function2/1 -> Add3/2
  Divide6/1 -> Divide7/1
  Add3/1 -> Divide10/1
  Constant21/1 -> Divide15/2
  Constant8/1 -> Divide6/1
  Add6/1 -> Divide15/1
  Constant22/1 -> Add6/1
  Divide11/1 -> Add4/2
  Divide10/1 -> Mh Static/1
  Divide7/1 -> Divide10/2
  Math Function/1 -> Add3/1
  Constant14/1 -> Divide8/1
  Divide8/1 -> Divide7/2
  Divide15/1 -> Math Function2/1
  Constant15/1 -> Add4/1
  Constant23/1 -> Add6/2
  Constant9/1 -> Divide6/2
  Constant16/1 -> Divide11/1
  Add4/1 -> Math Function/1
  Constant10/1 -> Divide6/3
  Constant11/1 -> Divide6/4
  Slip/1 -> Divide11/2, Divide8/2

== system model_vec/ASM1/Slip ==
  omega : Inport
  Add2 : Sum  Inputs=+-
  Constant12 : Constant  Value=2*pi*f
  Constant13 : Constant  Value=2*pi*f
  Divide9 : Product  Inputs=*/
  Slip : Outport
  wires:
  Constant13/1 -> Divide9/2
  Add2/1 -> Divide9/1
  Constant12/1 -> Add2/1
  Divide9/1 -> Slip/1
  omega/1 -> Add2/2  "Omega"

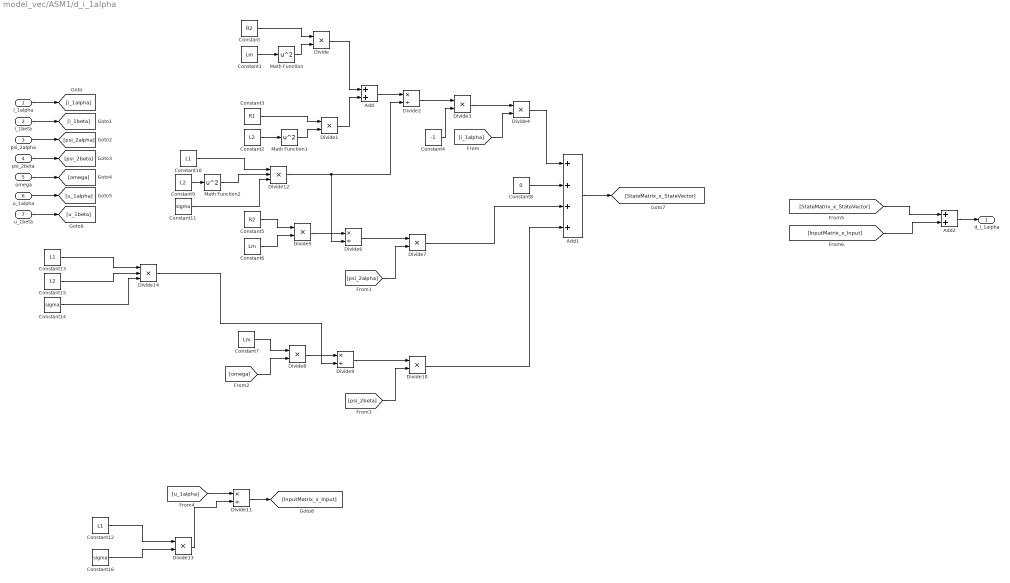
== system model_vec/ASM1/d_i_1alpha ==
  i_1alpha : Inport
  i_1beta : Inport  Port=2
  psi_2alpha : Inport  Port=3
  psi_2beta : Inport  Port=4
  omega : Inport  Port=5
  u_1alpha : Inport  Port=6
  u_1beta : Inport  Port=7
  Add : Sum
  Add1 : Sum  Inputs=++++
  Add2 : Sum
  Constant : Constant  Value=R2
  Constant1 : Constant  Value=Lm
  Constant10 : Constant  Value=L1
  Constant11 : Constant  Value=sigma
  Constant12 : Constant  Value=L1
  Constant13 : Constant  Value=L1
  Constant14 : Constant  Value=sigma
  Constant15 : Constant  Value=L2
  Constant16 : Constant  Value=sigma
  Constant2 : Constant  Value=L2
  Constant3 : Constant  Value=R1
  Constant4 : Constant  Value=-1
  Constant5 : Constant  Value=R2
  Constant6 : Constant  Value=Lm
  Constant7 : Constant  Value=Lm
  Constant8 : Constant  Value=0
  Constant9 : Constant  Value=L2
  Divide{,1,3..5,7..8,10,13} (9 alike) : Product  Inputs=**
  Divide{2,6,9,11} (4 alike) : Product  Inputs=*/
  Divide12 : Product  Inputs=***
  Divide14 : Product  Inputs=***
  Math Function : Math  Operator=square
  Math Function1 : Math  Operator=square
  Math Function2 : Math  Operator=square
  d_i_1alpha : Outport
  wires:
  Divide14/1 -> Divide9/2
  Divide13/1 -> Divide11/2
  Constant16/1 -> Divide13/2
  Constant12/1 -> Divide13/1
  Constant15/1 -> Divide14/2
  Constant13/1 -> Divide14/1
  Constant14/1 -> Divide14/3
  Divide12/1 -> Divide2/2, Divide6/2
  Constant11/1 -> Divide12/3
  Math Function2/1 -> Divide12/2
  Constant10/1 -> Divide12/1
  Constant9/1 -> Math Function2/1
  Add2/1 -> d_i_1alpha/1
  [InputMatrix_x_Input] -> Add2/2
  [StateMatrix_x_StateVector] -> Add2/1
  Divide11/1 -> [InputMatrix_x_Input]
  [u_1alpha] -> Divide11/1
  Add1/1 -> [StateMatrix_x_StateVector]
  u_1beta/1 -> [u_1beta]
  u_1alpha/1 -> [u_1alpha]
  Constant8/1 -> Add1/2
  Divide10/1 -> Add1/4
  [psi_2beta] -> Divide10/2
  Divide9/1 -> Divide10/1
  Divide8/1 -> Divide9/1
  [omega] -> Divide8/2
  Constant7/1 -> Divide8/1
  Divide7/1 -> Add1/3
  [psi_2alpha] -> Divide7/2
  Divide6/1 -> Divide7/1
  Divide5/1 -> Divide6/1
  Constant6/1 -> Divide5/2
  Constant5/1 -> Divide5/1
  Divide4/1 -> Add1/1
  [i_1alpha] -> Divide4/2
  omega/1 -> [omega]
  psi_2beta/1 -> [psi_2beta]
  psi_2alpha/1 -> [psi_2alpha]
  i_1beta/1 -> [i_1beta]
  i_1alpha/1 -> [i_1alpha]
  Divide3/1 -> Divide4/1
  Divide2/1 -> Divide3/1
  Constant4/1 -> Divide3/2
  Add/1 -> Divide2/1
  Divide1/1 -> Add/2
  Math Function1/1 -> Divide1/2
  Constant3/1 -> Divide1/1
  Constant2/1 -> Math Function1/1
  Divide/1 -> Add/1
  Math Function/1 -> Divide/2
  Constant/1 -> Divide/1
  Constant1/1 -> Math Function/1

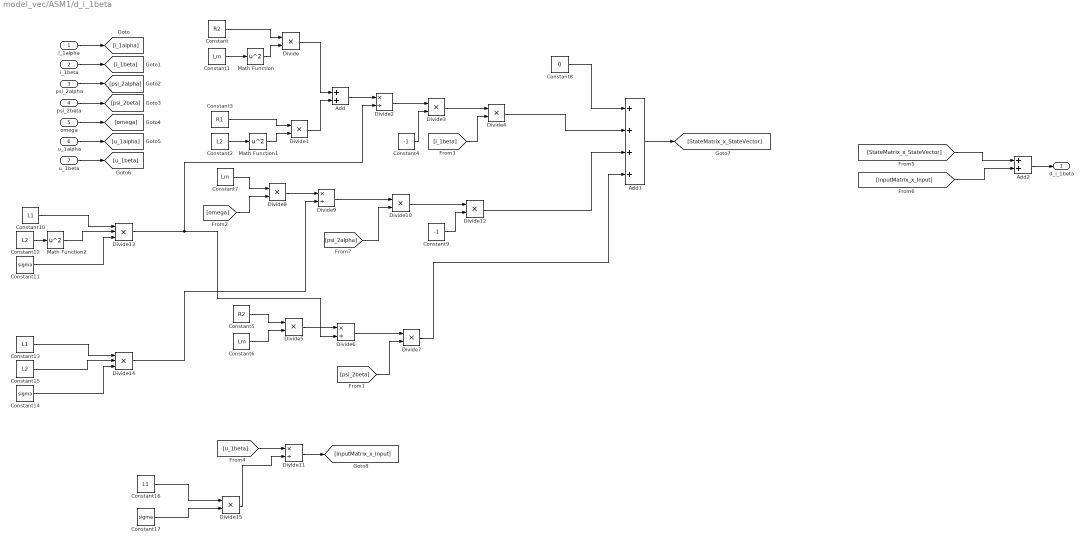
== system model_vec/ASM1/d_i_1beta ==
  i_1alpha : Inport
  i_1beta : Inport  Port=2
  psi_2alpha : Inport  Port=3
  psi_2beta : Inport  Port=4
  omega : Inport  Port=5
  u_1alpha : Inport  Port=6
  u_1beta : Inport  Port=7
  Add : Sum
  Add1 : Sum  Inputs=++++
  Add2 : Sum
  Constant : Constant  Value=R2
  Constant1 : Constant  Value=Lm
  Constant10 : Constant  Value=L1
  Constant11 : Constant  Value=sigma
  Constant12 : Constant  Value=L2
  Constant13 : Constant  Value=L1
  Constant14 : Constant  Value=sigma
  Constant15 : Constant  Value=L2
  Constant16 : Constant  Value=L1
  Constant17 : Constant  Value=sigma
  Constant2 : Constant  Value=L2
  Constant3 : Constant  Value=R1
  Constant4 : Constant  Value=-1
  Constant5 : Constant  Value=R2
  Constant6 : Constant  Value=Lm
  Constant7 : Constant  Value=Lm
  Constant8 : Constant  Value=0
  Constant9 : Constant  Value=-1
  Divide{,1,3..5,7..8,10,12,15} (10 alike) : Product  Inputs=**
  Divide{2,6,9,11} (4 alike) : Product  Inputs=*/
  Divide13 : Product  Inputs=***
  Divide14 : Product  Inputs=***
  Math Function : Math  Operator=square
  Math Function1 : Math  Operator=square
  Math Function2 : Math  Operator=square
  d_i_1beta : Outport
  wires:
  Constant17/1 -> Divide15/2
  Divide15/1 -> Divide11/2
  Constant16/1 -> Divide15/1
  Constant13/1 -> Divide14/1
  Constant15/1 -> Divide14/2
  Constant14/1 -> Divide14/3
  Divide14/1 -> Divide9/2
  Constant12/1 -> Math Function2/1
  Divide13/1 -> Divide2/2, Divide6/2
  Math Function2/1 -> Divide13/2
  Constant11/1 -> Divide13/3
  Constant10/1 -> Divide13/1
  Divide12/1 -> Add1/3
  Constant9/1 -> Divide12/2
  Constant1/1 -> Math Function/1
  Constant/1 -> Divide/1
  Math Function/1 -> Divide/2
  Divide/1 -> Add/1
  Constant2/1 -> Math Function1/1
  Constant3/1 -> Divide1/1
  Math Function1/1 -> Divide1/2
  Divide1/1 -> Add/2
  Add/1 -> Divide2/1
  Constant4/1 -> Divide3/2
  Divide2/1 -> Divide3/1
  Divide3/1 -> Divide4/1
  i_1alpha/1 -> [i_1alpha]
  i_1beta/1 -> [i_1beta]
  psi_2alpha/1 -> [psi_2alpha]
  psi_2beta/1 -> [psi_2beta]
  omega/1 -> [omega]
  [i_1beta] -> Divide4/2
  Divide4/1 -> Add1/2
  Constant5/1 -> Divide5/1
  Constant6/1 -> Divide5/2
  Divide5/1 -> Divide6/1
  Divide6/1 -> Divide7/1
  [psi_2beta] -> Divide7/2
  Divide7/1 -> Add1/4
  Constant7/1 -> Divide8/1
  [omega] -> Divide8/2
  Divide8/1 -> Divide9/1
  Divide9/1 -> Divide10/1
  [psi_2alpha] -> Divide10/2
  Divide10/1 -> Divide12/1
  Constant8/1 -> Add1/1
  u_1alpha/1 -> [u_1alpha]
  u_1beta/1 -> [u_1beta]
  Add1/1 -> [StateMatrix_x_StateVector]
  [u_1beta] -> Divide11/1
  Divide11/1 -> [InputMatrix_x_Input]
  [StateMatrix_x_StateVector] -> Add2/1
  [InputMatrix_x_Input] -> Add2/2
  Add2/1 -> d_i_1beta/1

== system model_vec/ASM1/d_psi_2alpha ==
  note: je to jen pro úplnost
  i_1alpha : Inport
  i_1beta : Inport  Port=2
  psi_2alpha : Inport  Port=3
  psi_2beta : Inport  Port=4
  omega : Inport  Port=5
  u_1alpha : Inport  Port=6
  u_1beta : Inport  Port=7
  Add1 : Sum  Inputs=++++
  Add2 : Sum
  Constant : Constant  Value=0
  Constant1 : Constant  Value=-1
  Constant2 : Constant  Value=-1
  Constant3 : Constant  Value=R2
  Constant4 : Constant  Value=L2
  Constant5 : Constant  Value=Lm
  Constant6 : Constant  Value=R2
  Constant7 : Constant  Value=L2
  Constant8 : Constant  Value=0
  Divide{,1,3..5,7} (6 alike) : Product  Inputs=**
  Divide2 : Product  Inputs=*/
  Divide6 : Product  Inputs=*/
  d_psi_2alpha : Outport
  wires:
  Divide7/1 -> Add1/1
  [i_1alpha] -> Divide7/2
  Divide6/1 -> Divide7/1
  Constant7/1 -> Divide6/2
  Constant6/1 -> Divide5/2
  Constant5/1 -> Divide5/1
  Divide5/1 -> Divide6/1
  Divide4/1 -> Add1/3
  [psi_2alpha] -> Divide4/2
  Divide3/1 -> Divide4/1
  Constant4/1 -> Divide2/2
  Constant3/1 -> Divide2/1
  Divide2/1 -> Divide3/1
  Constant2/1 -> Divide3/2
  Divide1/1 -> Add1/4
  [psi_2beta] -> Divide1/2
  Divide/1 -> Divide1/1
  Constant1/1 -> Divide/2
  [omega] -> Divide/1
  Add2/1 -> d_psi_2alpha/1
  [InputMatrix_x_Input] -> Add2/2
  [StateMatrix_x_StateVector] -> Add2/1
  Constant/1 -> [InputMatrix_x_Input]
  Add1/1 -> [StateMatrix_x_StateVector]
  u_1beta/1 -> [u_1beta]
  u_1alpha/1 -> [u_1alpha]
  Constant8/1 -> Add1/2
  omega/1 -> [omega]
  psi_2beta/1 -> [psi_2beta]
  psi_2alpha/1 -> [psi_2alpha]
  i_1beta/1 -> [i_1beta]
  i_1alpha/1 -> [i_1alpha]

== system model_vec/ASM1/d_psi_2beta ==
  i_1alpha : Inport
  i_1beta : Inport  Port=2
  psi_2alpha : Inport  Port=3
  psi_2beta : Inport  Port=4
  omega : Inport  Port=5
  u_1alpha : Inport  Port=6
  u_1beta : Inport  Port=7
  Add1 : Sum  Inputs=++++
  Add2 : Sum
  Constant : Constant  Value=0
  Constant2 : Constant  Value=-1
  Constant3 : Constant  Value=R2
  Constant4 : Constant  Value=L2
  Constant5 : Constant  Value=Lm
  Constant6 : Constant  Value=R2
  Constant7 : Constant  Value=L2
  Constant8 : Constant  Value=0
  Divide{1,3..5,7} (5 alike) : Product  Inputs=**
  Divide2 : Product  Inputs=*/
  Divide6 : Product  Inputs=*/
  d_psi_2beta : Outport
  wires:
  [omega] -> Divide1/1
  i_1alpha/1 -> [i_1alpha]
  i_1beta/1 -> [i_1beta]
  psi_2alpha/1 -> [psi_2alpha]
  psi_2beta/1 -> [psi_2beta]
  omega/1 -> [omega]
  Constant8/1 -> Add1/1
  u_1alpha/1 -> [u_1alpha]
  u_1beta/1 -> [u_1beta]
  Add1/1 -> [StateMatrix_x_StateVector]
  Constant/1 -> [InputMatrix_x_Input]
  [StateMatrix_x_StateVector] -> Add2/1
  [InputMatrix_x_Input] -> Add2/2
  Add2/1 -> d_psi_2beta/1
  [psi_2alpha] -> Divide1/2
  Divide1/1 -> Add1/3
  Constant2/1 -> Divide3/2
  Divide2/1 -> Divide3/1
  Constant3/1 -> Divide2/1
  Constant4/1 -> Divide2/2
  Divide3/1 -> Divide4/1
  [psi_2beta] -> Divide4/2
  Divide4/1 -> Add1/4
  Divide5/1 -> Divide6/1
  Constant5/1 -> Divide5/1
  Constant6/1 -> Divide5/2
  Constant7/1 -> Divide6/2
  Divide6/1 -> Divide7/1
  [i_1beta] -> Divide7/2
  Divide7/1 -> Add1/2
